simulink model "top_system"  (R2020b)
settings: Solver=ode15s  StartTime=0.0  StopTime=100  FixedStep=0.1  RelTol=1e-3
StartFcn:
  | fprintf(['Begin @ ' datestr(now,'HH:MM:SS\n')])
StopFcn:
  | fprintf(['Stop @ ' datestr(now,'HH:MM:SS\n')])
libraries: SignalEditorBlockLib x1, pid_lib x1
settings Model: Creator=jclinton  LastModifiedBy=jclinton
settings SolverCC: SolverJacobianMethodControl=SparseAnalytical
settings DataIOCC: SaveFormat=Array
settings DebuggingCC: SFMachineParentedDataDiag=error

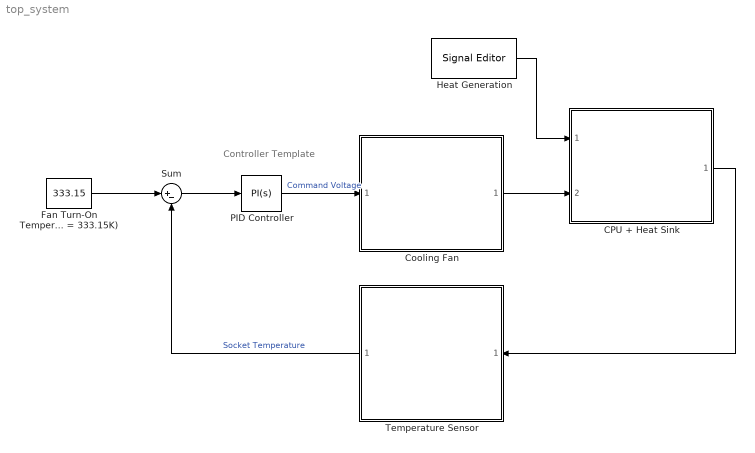
== system top_system ==
  note: Controller Template
  CPU + Heat Sink : Subsystem  ReferencedSubsystem=heat_sink  fidelityPARAM=Reduced Order Model  freqPARAM=[-Inf 20]  kPARAM=64
  Cooling Fan : Subsystem  ReferencedSubsystem=fan
  Fan Turn-On Temperature (60.0C = 333.15K) : Constant  Value=333.15
  Heat Generation : SignalEditorBlockLib/Signal Editor  FileName=HeatInput.mat  ActiveScenario=Scenario1  ActiveSignal=step20  IsBus=off  OutputBusObjectStr=Bus: BusObject  SampleTime=0  Interpolate=off  ZeroCross=off  OutputAfterFinalValue=Setting to zero  Unit=inherit  PreserveSignalName=on
  PID Controller : pid_lib/PID Controller  Controller=PI  Form=Parallel  TimeDomain=Continuous-time  UseExternalTs=off  SampleTime=-1  IntegratorMethod=Forward Euler  FilterMethod=Forward Euler  ControllerParametersSource=internal  P=-2  I=-0.1  D=0.5  UseFilter=on  N=100  TunerSelectOption=Transfer Function Based (PID Tuner App)  InitialConditionSource=internal  InitialConditionForIntegrator=0  InitialConditionForFilter=0  DifferentiatorICPrevScaledInput=0  ExternalReset=none  TrackingMode=off  Kt=1  LimitOutput=on  SatLimitsSource=internal  UpperSaturationLimit=12  LowerSaturationLimit=0  LinearizeAsGain=off  AntiWindupMode=clamping  Kb=1  POutMin=[]  POutMax=[]  IOutMin=[]  IOutMax=[]  DOutMin=[]  DOutMax=[]  NOutMin=[]  NOutMax=[]  SumOutMin=[]  SumOutMax=[]  SaturationOutMin=[]  SaturationOutMax=[]  PParamMin=[]  PParamMax=[]  IParamMin=[]  IParamMax=[]  DParamMin=[]  DParamMax=[]  NParamMin=[]  NParamMax=[]  KbParamMin=[]  KbParamMax=[]  KtParamMin=[]  KtParamMax=[]  KbOutMin=[]  KbOutMax=[]  KtOutMin=[]  KtOutMax=[]  IntegratorOutMin=[]  IntegratorOutMax=[]  FilterOutMin=[]  FilterOutMax=[]  SumI1OutMin=[]  SumI1OutMax=[]  SumI2OutMin=[]  SumI2OutMax=[]  SumI3OutMin=[]  SumI3OutMax=[]  SumI4OutMin=[]  SumI4OutMax=[]  SumDOutMin=[]  SumDOutMax=[]  DifferentiatorOutMin=[]  DifferentiatorOutMax=[]  FilterDiffOutCoefMin=[]  FilterDiffOutCoefMax=[]  ReciprocalOutMin=[]  ReciprocalOutMax=[]  SumDenOutMin=[]  SumDenOutMax=[]  SumNumOutMin=[]  SumNumOutMax=[]  DivideOutMin=[]  DivideOutMax=[]  UdiffTsProdOutMin=[]  UdiffTsProdOutMax=[]  NTsProdOutMin=[]  NTsProdOutMax=[]  UintegralTsProdOutMin=[]  UintegralTsProdOutMax=[]  UngainTsProdOutMin=[]  UngainTsProdOutMax=[]  IntegratorContinuousStateAttributes=''  IntegratorStateMustResolveToSignalObject=off  IntegratorRTWStateStorageClass=Auto  FilterContinuousStateAttributes=''  FilterStateMustResolveToSignalObject=off  FilterRTWStateStorageClass=Auto  ParallelPVariant=InternalParameters  IdealPVariant=Disabled  IVariant=InternalParameters  DVariant=Disabled  IntegratorVariant=Continuous  SatVariant=Enabled  AWVariant=ContClampingParallel  PCopyVariant=Disabled  TRVariant=Disabled  FdbkBlocksVariant=Forward  IdealPFdbkVariant=Disabled  SatFdbkVariant=Disabled  DerivativeFilterVariant=Disabled  NVariant=Disabled  NCopyVariant=Disabled_SignalSpec  FilterICVariant=Disabled  IntegratorICVariant=InternalICs  ExternalResetVariant=Disabled  TRSumVariant=Passthrough  SumFdbkVariant=Disabled  SumVariant=Sum_PI  TsampFilterVariant=InternalTs  TsampNgainVariant=Passthrough  TsampIntegralVariant=Passthrough  ExternalSaturationOutDataTypeStr=Inherit: Same as second input
  Sum : Sum  Inputs=|+-
  Temperature Sensor : Subsystem  ReferencedSubsystem=sensor
  wires:
  Sum/1 -> PID Controller/1
  Fan Turn-On Temperature (60.0C = 333.15K)/1 -> Sum/1
  PID Controller/1 -> Cooling Fan/1  "Command Voltage"
  Cooling Fan/1 -> CPU + Heat Sink/2
  CPU + Heat Sink/1 -> Temperature Sensor/1
  Temperature Sensor/1 -> Sum/2  "Socket Temperature"
  Heat Generation/1 -> CPU + Heat Sink/1
